simulink model "xobserver"  (R2018a)
settings: Solver=ode45  StartTime=0.0  StopTime=24.5344
model workspace (MAT data in the model file):
  control : struct (value not decoded)
  input : struct (value not decoded)
  l = 3335
  l1 = 2807
  l2 = 674
  lcontrol = 334
  lt = 665
  output : struct (value not decoded)
  output1 : struct (value not decoded)
  pitch = [-0.00601170594305 0.00114522514384 0.0125445164557 0.0260129427859 0.0413526501937 0.0511756269945 0.0373024628261 0.0532548324432 0.0752374412467 0.0870367972512 0.0703790408797 0.0642023494021 ... (665 elements, 665x1)]
  pitch1 = [0.00235222572609 0.0162413418271 0.0237914073903 0.038703711523 0.0528926975341 0.0693959637901 0.125700648169 0.149036541994 0.168586162345 0.181978559157 0.17648303704 0.173940572128 ... (665 elements, 665x1)]
  roll = [-0.00280308900026 -0.0093555701281 -0.00623960724973 -0.00965013944258 -0.0144960083544 -0.0165739618303 -0.0413451111402 -0.0417587932814 -0.039753610855 -0.0382742391951 -0.0474672160662 -0.0523524236581 ... (665 elements, 665x1)]
  roll1 = [-0.00508976540984 -0.0128769177256 -0.00573808802069 -0.00803683640664 -0.0148569990238 -0.0135250113299 0.00757283220458 0.0108108566268 0.0110824245139 0.0117467287189 0.0115391118445 0.00812049366445 ... (665 elements, 665x1)]
  rtk_P = [0 0 0.00725817699424 0.00725817699424 -4.192609801e-16 -4.192609801e-16 0.00725817698288 0.00725817698288 -6.06069014419e-17 -6.06069014419e-17 0.00725817697152 0.00725817697152 ... (2022 elements, 674x3)]
  simin : struct (value not decoded)
  t = [85.2681087899 153.847078989 135.937655107 145.710208503 139.738803374 143.646452387 141.245887466 142.795164057 141.986419874 142.477492231 142.340892456 142.389396391 ... (674 elements, 674x1)]
  temp = [0.000186264650653 -0.000333016556148 0.00127742410264 0.00224038281138 0.00429726594319 -0.00123745127094 -0.0498635877438 -0.0654781132175 -0.0797628012916 -0.0994190421594 -0.130389530625 -0.157448428987 ... (674 elements, 674x1)]
  time = [137013148 137105522 137113114 137205498 137213142 137305502 137313143 137385536 137393177 137505497 137513125 137605502 ... (665 elements, 665x1)]
  tout = [0 40 80 120 160 200 240 280 320 360 400 440 ... (51 elements, 51x1)]
  ups = [-0.00390798864963 -0.0343320965106 -0.0636578539957 -0.075087173802 -0.0805963166531 -0.0991310672402 -0.125807682301 -0.141612416937 -0.141039897482 -0.132345709554 -0.120718475957 -0.105525554245 ... (665 elements, 665x1)]
  urs = [-0.0193064957453 -0.00988556947443 0.00896900324588 0.0192245887848 0.0131872654637 -0.000864770461033 -0.0106332547779 -0.00981483295256 -0.00119475892361 0.00693320512295 0.00799889781381 0.00317561720843 ... (665 elements, 665x1)]
  uts = [0.664106860951 0.749481484877 0.672099541838 0.648171853238 0.700691335264 0.708512249166 0.659850468498 0.640879189244 0.664961763399 0.668205140062 0.640989688844 0.625700347079 ... (665 elements, 665x1)]
  uys = [0.0139395447601 0.0198481563309 0.0256425224772 0.0339606547853 0.0446716994275 0.0544470884218 0.06301463774 0.0718767917399 0.0826736407 0.0943232231429 0.10641126735 0.11853603151 ... (665 elements, 665x1)]
  x = [8.71560944851e-05 -0.000263895544732 0.000265805954332 0.000300014003894 0.000591371497193 0.000529778841884 0.00684193504836 0.00668914061072 0.00254694811157 -0.00143805981445 -0.0136823182856 -0.0178010839904 ... (665 elements, 665x1)]
  x1 = [8.54283814042e-05 -0.000351541918258 0.000561343727981 0.00122062991294 0.00226118745505 0.0017878063312 -0.0048216263535 -0.0106732543262 -0.0180693220189 -0.0278330591582 -0.0298109986026 -0.0413157469741 ... (665 elements, 665x1)]
  x_av = [8.62922379446e-05 -0.000307718731495 0.000413574841157 0.000760321958416 0.00142627947612 0.00115879258654 0.00101015434743 -0.00199205685772 -0.00776118695365 -0.0146355594863 -0.0217466584441 -0.0295584154823 ... (665 elements, 665x1)]
  xt = [-6.06069014419e-17 0.00725817697152 0.00725817697152 -5.47955244547e-11 -5.47955244547e-11 -5.57118682784e-11 -5.57118682784e-11 -0.00725817702815 -0.00725817702815 -0.0145163542274 -0.0145163542274 -0.0290327088019 ... (665 elements, 665x1)]
  y = [4.71199364932e-05 -0.000202451032641 0.00110205359743 0.00274075291804 0.00386317545071 0.0039759501557 0.0111320604636 0.0200674919449 0.0256167559869 0.0328388617799 0.00902856975366 0.0187732326011 ... (665 elements, 665x1)]
  y1 = [0.000186264650653 -0.000333016556148 0.00127742410264 0.00224038281138 0.00429726594319 -0.00123745127094 -0.0498635877438 -0.0654781132175 -0.0797628012916 -0.0994190421594 -0.130389530625 -0.157448428987 ... (665 elements, 665x1)]
  y_av = [0.000116692293573 -0.000267733794395 0.00118973885004 0.00249056786471 0.00408022069695 0.00136924944238 -0.0193657636401 -0.0227053106363 -0.0270730226523 -0.0332900901898 -0.0606804804357 -0.0693375981928 ... (665 elements, 665x1)]
  yaw = [0.551630744054 0.985953522054 0.860467849076 0.912170384354 0.864267212524 0.877979115519 0.85252446167 0.850917442274 0.835099319744 0.825993656962 0.8192363021 0.809230396231 ... (665 elements, 665x1)]
  yaw1 = [0.524311158471 0.914078236382 0.795656408279 0.841193934159 0.796803282272 0.809519389357 0.787366234758 0.785910630038 0.771945888619 0.763168855651 0.757543515422 0.745155737898 ... (665 elements, 665x1)]
  yt = [2.07646400074e-15 -8.22783768201e-10 -8.22783768201e-10 -0.0111218847698 -0.0111218847698 -0.0222437696223 -0.0222437696223 -0.0333656546197 -0.0333656546197 -0.0444875400883 -0.0444875400883 -0.0667313107556 ... (665 elements, 665x1)]
  z = [-0.0994666679592 -0.214162644666 -0.215226967159 -0.256145303395 -0.292239651406 -0.309925352113 -0.350361829325 -0.36096245045 -0.394865238248 -0.398678408621 -0.417742992449 -0.417553654594 ... (674 elements, 674x1)]
  z1 = [-0.103229820714 -0.203136396463 -0.194407590044 -0.247819005734 -0.277075354685 -0.291884441153 -0.321788426104 -0.334001860067 -0.367445284083 -0.368818531247 -0.415153871284 -0.416306471083 ... (674 elements, 674x1)]
libraries: dspmathops x3
(part 2 of 2)

== system xobserver/Norm 1 ==
  In1 : Inport
  In2 : Inport  Port=2
  Sqrt : Sqrt  SaturateOnIntegerOverflow=on
  Square : Math  Operator=square  SaturateOnIntegerOverflow=on
  Square1 : Math  Operator=square  SaturateOnIntegerOverflow=on
  Sum2 : Sum  Inputs=|++
  Out1 : Outport
  wires:
  Sum2/1 -> Sqrt/1
  Square1/1 -> Sum2/2
  Square/1 -> Sum2/1
  In2/1 -> Square1/1
  Sqrt/1 -> Out1/1
  In1/1 -> Square/1

== system xobserver/Norm 2 ==
  In1 : Inport
  In2 : Inport  Port=2
  Sqrt : Sqrt  SaturateOnIntegerOverflow=on
  Square : Math  Operator=square  SaturateOnIntegerOverflow=on
  Square1 : Math  Operator=square  SaturateOnIntegerOverflow=on
  Sum2 : Sum  Inputs=|++
  Out1 : Outport
  wires:
  Sum2/1 -> Sqrt/1
  Square1/1 -> Sum2/2
  Square/1 -> Sum2/1
  In2/1 -> Square1/1
  Sqrt/1 -> Out1/1
  In1/1 -> Square/1

== system xobserver/Norm 3 ==
  In1 : Inport
  In2 : Inport  Port=2
  Sqrt : Sqrt  SaturateOnIntegerOverflow=on
  Square : Math  Operator=square  SaturateOnIntegerOverflow=on
  Square1 : Math  Operator=square  SaturateOnIntegerOverflow=on
  Sum2 : Sum  Inputs=|++
  Out1 : Outport
  wires:
  Sum2/1 -> Sqrt/1
  Square1/1 -> Sum2/2
  Square/1 -> Sum2/1
  In2/1 -> Square1/1
  Sqrt/1 -> Out1/1
  In1/1 -> Square/1

== system xobserver/Norm 5 ==
  In1 : Inport
  In2 : Inport  Port=2
  Sqrt : Sqrt  SaturateOnIntegerOverflow=on
  Square : Math  Operator=square  SaturateOnIntegerOverflow=on
  Square1 : Math  Operator=square  SaturateOnIntegerOverflow=on
  Sum2 : Sum  Inputs=|++
  Out1 : Outport
  wires:
  Sum2/1 -> Sqrt/1
  Square1/1 -> Sum2/2
  Square/1 -> Sum2/1
  In2/1 -> Square1/1
  Sqrt/1 -> Out1/1
  In1/1 -> Square/1

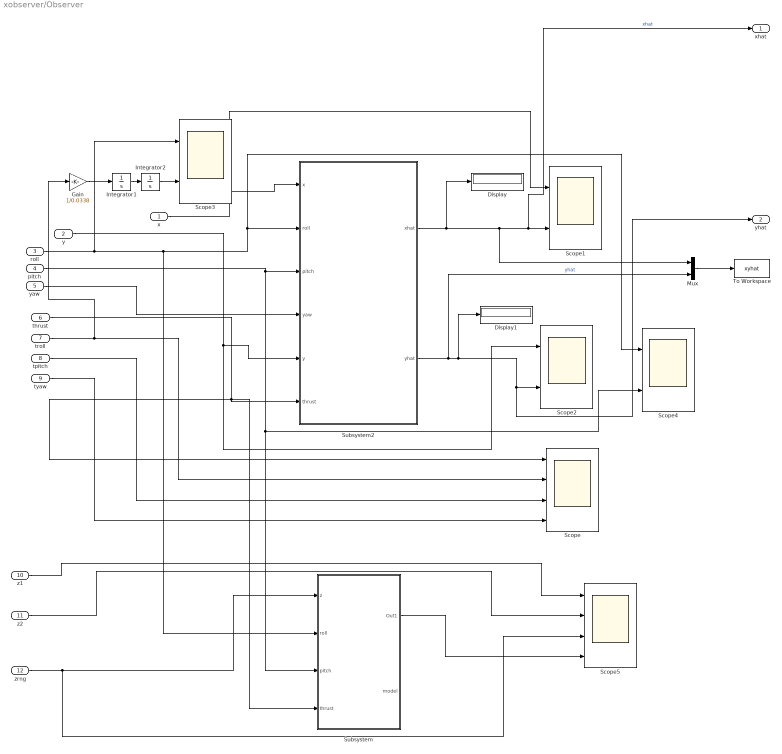
== system xobserver/Observer  ==
  x : Inport
  y : Inport  Port=2
  roll : Inport  Port=3
  pitch : Inport  Port=4
  yaw : Inport  Port=5
  thrust : Inport  Port=6
  troll : Inport  Port=7
  tpitch : Inport  Port=8
  tyaw : Inport  Port=9
  z1 : Inport  Port=10
  z2 : Inport  Port=11
  "zrng " : Inport  Port=12
  Display : Display
  Display1 : Display
  Gain : Gain  Gain=1/0.0338
  Integrator1 : Integrator
  Integrator2 : Integrator
  Mux : Mux  Inputs=2
  Scope : Scope  NumInputPorts=4
  Scope{1..4} (4 alike) : Scope  NumInputPorts=2
  Scope5 : Scope  NumInputPorts=4
  Subsystem : Subsystem
  Subsystem2 : Subsystem
  To Workspace : ToWorkspace  VariableName=xyhat  SampleTime=0.01
  xhat : Outport
  yhat : Outport  Port=2
  wires:
  y/1 -> Subsystem2/5(y), Scope2/1
  pitch/1 -> Scope4/2, Subsystem/3(pitch), Subsystem2/3(pitch)
  tyaw/1 -> Scope/4
  Subsystem2/2(yhat) -> Mux/2, Display1/1, yhat/1, Scope2/2  "yhat"
  thrust/1 -> Scope/1, Subsystem2/6(thrust), Subsystem/4(thrust)
  roll/1 -> Scope4/1, Subsystem2/2(roll), Subsystem/2(roll), Scope3/1
  troll/1 -> Gain/1, Scope/2
  Mux/1 -> To Workspace/1
  x/1 -> Subsystem2/1(x), Scope1/1
  yaw/1 -> Subsystem2/4(yaw)
  tpitch/1 -> Scope/3
  Gain/1 -> Integrator1/1
  Integrator1/1 -> Integrator2/1
  Integrator2/1 -> Scope3/2
  Subsystem2/1(xhat) -> Display/1, xhat/1, Scope1/2, Mux/1  "xhat"
  z1/1 -> Scope5/1
  z2/1 -> Scope5/2
  "zrng "/1 -> Subsystem/1(z), Scope5/3
  Subsystem/1(Out1) -> Scope5/4

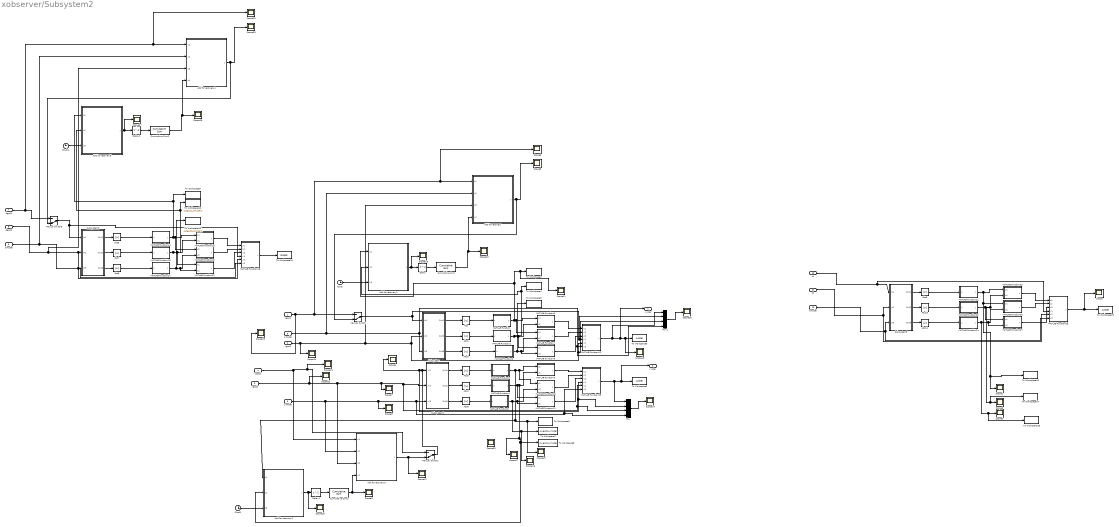
== system xobserver/Subsystem2 ==
  "xgps1 " : Inport
  "xgps2 " : Inport  Port=2
  "ygps2 " : Inport  Port=3
  ygps1 : Inport  Port=4
  "xmodel " : Inport  Port=5
  "ymodel " : Inport  Port=6
  "dgps1 " : Inport  Port=7
  dgps2 : Inport  Port=8
  "dmodel " : Inport  Port=9
  "z1 " : Inport  Port=10
  z2 : Inport  Port=11
  "zmodel " : Inport  Port=12
  Abs{,1..11} (12 alike) : Abs
  Add for recovery : MATLAB Function  TreatAsAtomicUnit=on
  Add for recovery1 : MATLAB Function  TreatAsAtomicUnit=on
  Add for recovery2 : MATLAB Function  TreatAsAtomicUnit=on
  Add for recovery3 : MATLAB Function  TreatAsAtomicUnit=on
  Add for recovery4 : MATLAB Function  TreatAsAtomicUnit=on
  Add for recovery5 : MATLAB Function  TreatAsAtomicUnit=on
  Clock : Clock
  Clock1 : Clock
  Clock2 : Clock
  Cumulative Sum : dspmathops/Cumulative Sum  dim=Channels (running sum)  InputProcessing=Columns as channels (frame based)  reset_popup=None  roundingMode=Floor  overflowMode=off  outputDataTypeStr=Inherit: Same as accumulator  outputMin=[]  outputMax=[]  outputLastDataTypeStr=Inherit: Same as accumulator
      settings: SourceProductName=DSP System Toolbox
  Cumulative Sum1 : dspmathops/Cumulative Sum  dim=Channels (running sum)  InputProcessing=Columns as channels (frame based)  reset_popup=None  roundingMode=Floor  overflowMode=off  outputDataTypeStr=Inherit: Same as accumulator  outputMin=[]  outputMax=[]  outputLastDataTypeStr=Inherit: Same as accumulator
      settings: SourceProductName=DSP System Toolbox
  Cumulative Sum2 : dspmathops/Cumulative Sum  dim=Channels (running sum)  InputProcessing=Columns as channels (frame based)  reset_popup=None  roundingMode=Floor  overflowMode=off  outputDataTypeStr=Inherit: Same as accumulator  outputMin=[]  outputMax=[]  outputLastDataTypeStr=Inherit: Same as accumulator
      settings: SourceProductName=DSP System Toolbox
  Delay : Delay
  Delay1 : Delay
  Delay2 : Delay
  MATLAB Function : MATLAB Function  TreatAsAtomicUnit=on
  MATLAB Function1 : MATLAB Function  TreatAsAtomicUnit=on
  MATLAB Function10 : MATLAB Function  TreatAsAtomicUnit=on
  MATLAB Function11 : MATLAB Function  TreatAsAtomicUnit=on
  MATLAB Function12 : MATLAB Function  TreatAsAtomicUnit=on
  MATLAB Function13 : MATLAB Function  TreatAsAtomicUnit=on
  MATLAB Function14 : MATLAB Function  TreatAsAtomicUnit=on
  MATLAB Function15 : MATLAB Function  TreatAsAtomicUnit=on
  MATLAB Function16 : MATLAB Function  TreatAsAtomicUnit=on
  MATLAB Function17 : MATLAB Function  TreatAsAtomicUnit=on
  MATLAB Function18 : MATLAB Function  TreatAsAtomicUnit=on
  MATLAB Function19 : MATLAB Function  TreatAsAtomicUnit=on
  MATLAB Function2 : MATLAB Function  TreatAsAtomicUnit=on
  MATLAB Function20 : MATLAB Function  TreatAsAtomicUnit=on
  MATLAB Function21 : MATLAB Function  TreatAsAtomicUnit=on
  MATLAB Function22 : MATLAB Function  TreatAsAtomicUnit=on
  MATLAB Function23 : MATLAB Function  TreatAsAtomicUnit=on
  MATLAB Function24 : MATLAB Function  TreatAsAtomicUnit=on
  MATLAB Function25 : MATLAB Function  TreatAsAtomicUnit=on
  MATLAB Function26 : MATLAB Function  TreatAsAtomicUnit=on
  MATLAB Function27 : MATLAB Function  TreatAsAtomicUnit=on
  MATLAB Function3 : MATLAB Function  TreatAsAtomicUnit=on
  MATLAB Function4 : MATLAB Function  TreatAsAtomicUnit=on
  MATLAB Function5 : MATLAB Function  TreatAsAtomicUnit=on
  MATLAB Function6 : MATLAB Function  TreatAsAtomicUnit=on
  MATLAB Function7 : MATLAB Function  TreatAsAtomicUnit=on
  MATLAB Function8 : MATLAB Function  TreatAsAtomicUnit=on
  MATLAB Function9 : MATLAB Function  TreatAsAtomicUnit=on
  Manual Switch : ManualSwitch  CurrentSetting=0
  Manual Switch1 : ManualSwitch  CurrentSetting=0
  Manual Switch3 : ManualSwitch  CurrentSetting=0
  Mux : Mux
  Mux1 : Mux
  Scope{,1..29} (30 alike) : Scope
  Subsystem : Subsystem
  Subsystem1 : Subsystem
  Subsystem2 : Subsystem
  Subsystem3 : Subsystem
  To Workspace1 : ToWorkspace  VariableName=yvoter  SampleTime=0.01
  To Workspace10 : ToWorkspace  VariableName=dvoter  SampleTime=0.01
  To Workspace11 : ToWorkspace  VariableName=s_dgps1_dmodel1  SampleTime=-1
  To Workspace12 : ToWorkspace  VariableName=s_dgps2_dmodel1  SampleTime=-1
  To Workspace13 : ToWorkspace  VariableName=zvoter  SampleTime=0.01
  To Workspace14 : ToWorkspace  VariableName=s_zrng1_zmodel  SampleTime=-1
  To Workspace15 : ToWorkspace  VariableName=s_zrng2_zmodel  SampleTime=-1
  To Workspace16 : ToWorkspace  VariableName=s_zrng1_zrng2  SampleTime=-1
  To Workspace2 : ToWorkspace  VariableName=s_xgps1_xgps2  SampleTime=-1
  To Workspace3 : ToWorkspace  VariableName=xvoter  SampleTime=0.01
  To Workspace4 : ToWorkspace  VariableName=s_xgps1_xmodel  SampleTime=-1
  To Workspace5 : ToWorkspace  VariableName=s_xgps2_xmodel  SampleTime=-1
  To Workspace6 : ToWorkspace  VariableName=s_ygps1_ygps2  SampleTime=-1
  To Workspace7 : ToWorkspace  VariableName=s_ygps2_ymodel  SampleTime=-1
  To Workspace8 : ToWorkspace  VariableName=s_ygps1_ymodel  SampleTime=-1
  To Workspace9 : ToWorkspace  VariableName=s_dgps1_dgps2  SampleTime=-1
  "xvoter " : Outport
  yvoter : Outport  Port=2
  wires:
  Subsystem/1(Out1) -> Abs/1
  Subsystem/3(Out3) -> Abs2/1
  "ymodel "/1 -> Add for recovery3/2(u2), Scope8/1, Subsystem1/3(In3), Mux/4, MATLAB Function13/6(x3)
  MATLAB Function9/1(y) -> MATLAB Function13/1(u1)
  MATLAB Function11/1(y) -> MATLAB Function13/3(u3)
  Manual Switch1/1 -> Scope4/1, Mux/2, MATLAB Function13/4(x1), Subsystem1/1(In1)
  Subsystem/2(Out2) -> Abs1/1
  Subsystem1/3(Out3) -> Abs5/1
  MATLAB Function4/1(y) -> Scope17/1, Add for recovery2/2(u2), To Workspace8/1, MATLAB Function9/2(u2), MATLAB Function11/1(u1)
  "xgps2 "/1 -> Scope24/1, Subsystem/2(In2), Mux1/3, MATLAB Function12/5(x2), Add for recovery/3(u3)
  MATLAB Function/1(y) -> Add for recovery1/1(u1), Scope11/1, To Workspace2/1, MATLAB Function7/1(u1), MATLAB Function6/1(u1)
  MATLAB Function2/1(y) -> To Workspace5/1, MATLAB Function8/2(u2), MATLAB Function7/2(u2)
  MATLAB Function13/1(y) -> Mux/1, yvoter/1, To Workspace1/1
  MATLAB Function5/1(y) -> MATLAB Function10/2(u2), MATLAB Function11/2(u2), Scope16/1, To Workspace7/1
  MATLAB Function3/1(y) -> Add for recovery2/1(u1), Scope15/1, To Workspace6/1, MATLAB Function10/1(u1), MATLAB Function9/1(u1)
  Manual Switch/1 -> Mux1/2, MATLAB Function12/4(x1), Subsystem/1(In1)
  MATLAB Function12/1(y) -> Mux1/1, "xvoter "/1, Scope13/1, To Workspace3/1
  MATLAB Function8/1(y) -> MATLAB Function12/3(u3)
  MATLAB Function1/1(y) -> Add for recovery1/2(u2), To Workspace4/1, MATLAB Function8/1(u1), MATLAB Function6/2(u2)
  "xmodel "/1 -> Add for recovery/2(u2), Subsystem/3(In3), Mux1/4, MATLAB Function12/6(x3)
  MATLAB Function7/1(y) -> MATLAB Function12/2(u2)
  MATLAB Function6/1(y) -> MATLAB Function12/1(u1)
  "ygps2 "/1 -> Scope22/1, Add for recovery3/3(u3), Scope7/1, Subsystem1/2(In2), Mux/3, MATLAB Function13/5(x2)
  Subsystem1/1(Out1) -> Abs3/1
  Subsystem1/2(Out2) -> Abs4/1
  MATLAB Function10/1(y) -> MATLAB Function13/2(u2)
  MATLAB Function18/1(y) -> MATLAB Function16/1(u1)
  MATLAB Function19/1(y) -> MATLAB Function16/2(u2)
  MATLAB Function16/1(y) -> To Workspace10/1
  MATLAB Function20/1(y) -> MATLAB Function16/3(u3)
  MATLAB Function15/1(y) -> Add for recovery5/2(u2), To Workspace11/1, MATLAB Function20/1(u1), MATLAB Function18/2(u2)
  MATLAB Function14/1(y) -> Add for recovery5/1(u1), To Workspace9/1, MATLAB Function19/1(u1), MATLAB Function18/1(u1)
  MATLAB Function17/1(y) -> To Workspace12/1, MATLAB Function20/2(u2), MATLAB Function19/2(u2)
  Subsystem2/1(Out1) -> Abs6/1
  Subsystem2/2(Out2) -> Abs7/1
  Subsystem2/3(Out3) -> Abs8/1
  Abs/1 -> MATLAB Function/1(u)
  Abs1/1 -> MATLAB Function1/1(u)
  Abs2/1 -> MATLAB Function2/1(u)
  Abs3/1 -> MATLAB Function3/1(u)
  Abs4/1 -> MATLAB Function4/1(u)
  Abs5/1 -> MATLAB Function5/1(u)
  Abs6/1 -> MATLAB Function14/1(u)
  Abs7/1 -> MATLAB Function15/1(u)
  Abs8/1 -> MATLAB Function17/1(u)
  MATLAB Function21/1(y) -> To Workspace16/1, Scope1/1, MATLAB Function26/1(u1), MATLAB Function25/1(u1)
  MATLAB Function24/1(y) -> To Workspace15/1, Scope3/1, MATLAB Function27/2(u2), MATLAB Function26/2(u2)
  Abs10/1 -> MATLAB Function22/1(u)
  Abs11/1 -> MATLAB Function24/1(u)
  Abs9/1 -> MATLAB Function21/1(u)
  MATLAB Function25/1(y) -> MATLAB Function23/1(u1)
  Subsystem3/2(Out2) -> Abs10/1
  MATLAB Function26/1(y) -> MATLAB Function23/2(u2)
  Subsystem3/1(Out1) -> Abs9/1
  MATLAB Function23/1(y) -> Scope/1, To Workspace13/1
  MATLAB Function27/1(y) -> MATLAB Function23/3(u3)
  MATLAB Function22/1(y) -> To Workspace14/1, Scope2/1, MATLAB Function25/2(u2), MATLAB Function27/1(u1)
  Subsystem3/3(Out3) -> Abs11/1
  "xgps1 "/1 -> Scope23/1, Scope6/1, Add for recovery/1(u1), Manual Switch/1
  Clock/1 -> Add for recovery1/3(u3)
  Clock1/1 -> Add for recovery2/3(u3)
  ygps1/1 -> Scope21/1, Manual Switch1/1, Add for recovery3/1(u1)
  Add for recovery1/1(y) -> Scope19/1, Delay/1
  Cumulative Sum/1 -> Add for recovery/4(u4), Scope10/1
  Delay/1 -> Cumulative Sum/1
  Delay1/1 -> Cumulative Sum1/1
  Add for recovery2/1(y) -> Scope18/1, Delay1/1
  Cumulative Sum1/1 -> Add for recovery3/4(u4), Scope9/1
  Add for recovery3/1(y) -> Scope12/1, Manual Switch1/2
  Add for recovery/1(y) -> Manual Switch/2, Scope5/1
  Mux/1 -> Scope14/1
  Mux1/1 -> Scope20/1
  z2/1 -> MATLAB Function23/5(x2), Subsystem3/2(In2)
  "zmodel "/1 -> MATLAB Function23/6(x3), Subsystem3/3(In3)
  "z1 "/1 -> MATLAB Function23/4(x1), Subsystem3/1(In1)
  dgps2/1 -> Add for recovery4/3(u3), MATLAB Function16/5(x2), Subsystem2/2(In2)
  "dmodel "/1 -> Add for recovery4/2(u2), MATLAB Function16/6(x3), Subsystem2/3(In3)
  "dgps1 "/1 -> Scope29/1, Add for recovery4/1(u1), Manual Switch3/1
  Add for recovery4/1(y) -> Manual Switch3/2, Scope28/1
  Cumulative Sum2/1 -> Add for recovery4/4(u4), Scope26/1
  Add for recovery5/1(y) -> Scope27/1, Delay2/1
  Delay2/1 -> Cumulative Sum2/1
  Clock2/1 -> Add for recovery5/3(u3)
  Manual Switch3/1 -> MATLAB Function16/4(x1), Subsystem2/1(In1)

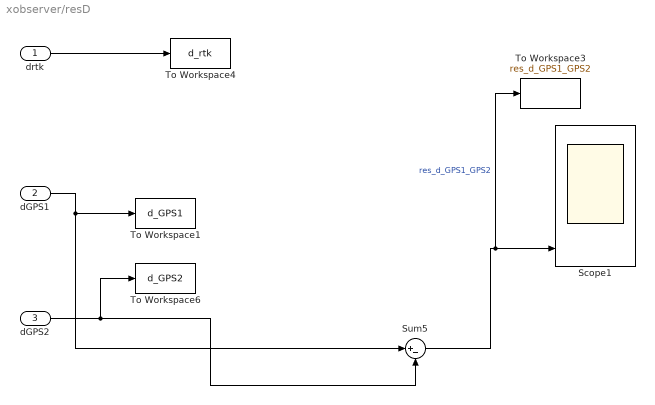
== system xobserver/resD ==
  drtk : Inport
  dGPS1 : Inport  Port=2
  dGPS2 : Inport  Port=3
  Scope1 : Scope  NumInputPorts=4
  Sum5 : Sum  Inputs=|+-
  To Workspace1 : ToWorkspace  VariableName=d_GPS1  SampleTime=0.01
  To Workspace3 : ToWorkspace  VariableName=res_d_GPS1_GPS2  SampleTime=0.01
  To Workspace4 : ToWorkspace  VariableName=d_rtk  SampleTime=0.01
  To Workspace6 : ToWorkspace  VariableName=d_GPS2  SampleTime=0.01
  wires:
  Sum5/1 -> To Workspace3/1, Scope1/4  "res_d_GPS1_GPS2"
  dGPS2/1 -> To Workspace6/1, Sum5/2
  drtk/1 -> To Workspace4/1
  dGPS1/1 -> To Workspace1/1, Sum5/1

== system xobserver/resD1 ==
  xrtk : Inport
  xGPS1 : Inport  Port=2
  xGPS2 : Inport  Port=3
  Scope1 : Scope  NumInputPorts=4
  Sum5 : Sum  Inputs=|+-
  To Workspace3 : ToWorkspace  VariableName=res_x_GPS1_GPS2  SampleTime=0.01
  wires:
  xGPS1/1 -> Sum5/1
  xGPS2/1 -> Sum5/2
  Sum5/1 -> To Workspace3/1, Scope1/4  "res_x_GPS1_GPS2"

== system xobserver/resD2 ==
  yrtk : Inport
  yGPS1 : Inport  Port=2
  yGPS2 : Inport  Port=3
  Scope1 : Scope  NumInputPorts=4
  Sum5 : Sum  Inputs=|+-
  To Workspace3 : ToWorkspace  VariableName=res_y_GPS1_GPS2  SampleTime=0.01
  wires:
  yGPS1/1 -> Sum5/1
  Sum5/1 -> To Workspace3/1, Scope1/4  "res_y_GPS1_GPS2"
  yGPS2/1 -> Sum5/2

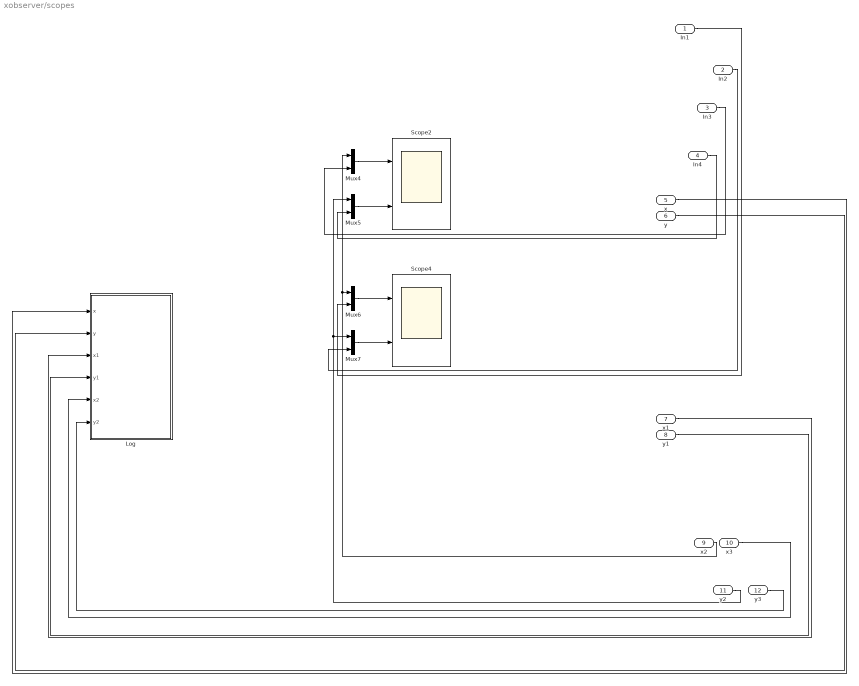
== system xobserver/scopes  ==
  In1 : Inport
  In2 : Inport  Port=2
  In3 : Inport  Port=3
  In4 : Inport  Port=4
  x : Inport  Port=5
  y : Inport  Port=6
  x1 : Inport  Port=7
  y1 : Inport  Port=8
  x2 : Inport  Port=9
  x3 : Inport  Port=10
  y2 : Inport  Port=11
  y3 : Inport  Port=12
  "Log " : Subsystem
  Mux{4..7} (4 alike) : Mux  Inputs=2
  Scope2 : Scope  NumInputPorts=2
  Scope4 : Scope  NumInputPorts=2
  wires:
  In3/1 -> Mux4/2
  In1/1 -> Mux6/2
  y1/1 -> "Log "/4(y1)
  Mux7/1 -> Scope4/2
  y2/1 -> Mux7/1, Mux5/1
  Mux6/1 -> Scope4/1
  Mux5/1 -> Scope2/2
  Mux4/1 -> Scope2/1
  x2/1 -> Mux6/1, Mux4/1
  In2/1 -> Mux7/2
  In4/1 -> Mux5/2
  y/1 -> "Log "/2(y)
  x/1 -> "Log "/1(x)
  x1/1 -> "Log "/3(x1)
  y3/1 -> "Log "/6(y2)
  x3/1 -> "Log "/5(x2)

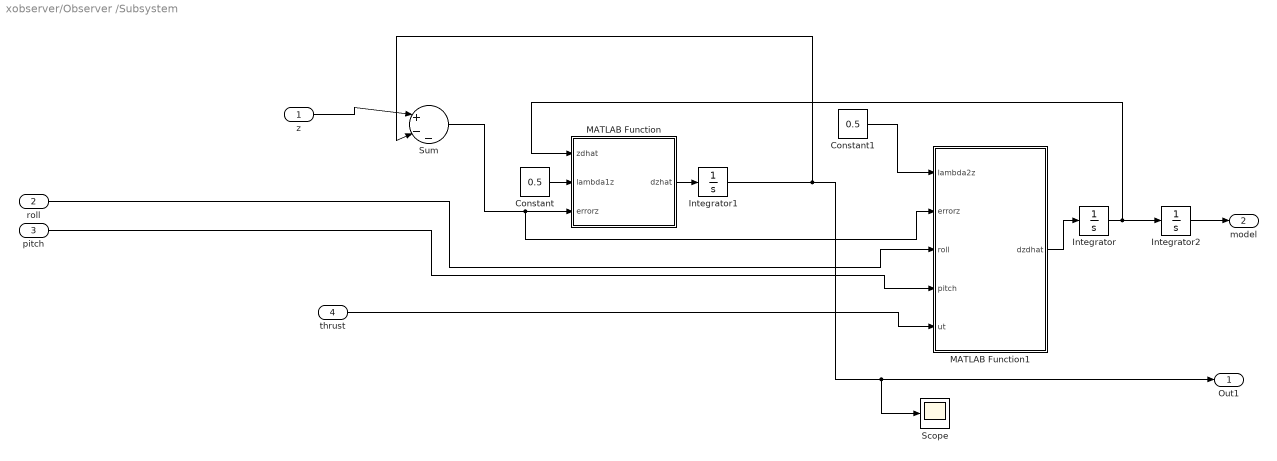
== system xobserver/Observer /Subsystem ==
  z : Inport
  roll : Inport  Port=2
  pitch : Inport  Port=3
  thrust : Inport  Port=4
  Constant : Constant  Value=0.5
  Constant1 : Constant  Value=0.5
  Integrator : Integrator  InitialCondition=0
  Integrator1 : Integrator  InitialCondition=0.1332
  Integrator2 : Integrator
  MATLAB Function : MATLAB Function  TreatAsAtomicUnit=on
  MATLAB Function1 : MATLAB Function  TreatAsAtomicUnit=on
  Scope : Scope
  Sum : Sum  Inputs=|+--
  Out1 : Outport
  "model " : Outport  Port=2
  wires:
  MATLAB Function/1(dzhat) -> Integrator1/1
  Integrator/1 -> Integrator2/1, MATLAB Function/1(zdhat)
  Constant1/1 -> MATLAB Function1/1(lambda2z)
  roll/1 -> MATLAB Function1/3(roll)
  Constant/1 -> MATLAB Function/2(lambda1z)
  MATLAB Function1/1(dzdhat) -> Integrator/1
  pitch/1 -> MATLAB Function1/4(pitch)
  thrust/1 -> MATLAB Function1/5(ut)
  z/1 -> Sum/1
  Integrator2/1 -> "model "/1
  Sum/1 -> MATLAB Function1/2(errorz), MATLAB Function/3(errorz)
  Integrator1/1 -> Sum/2, Scope/1, Out1/1

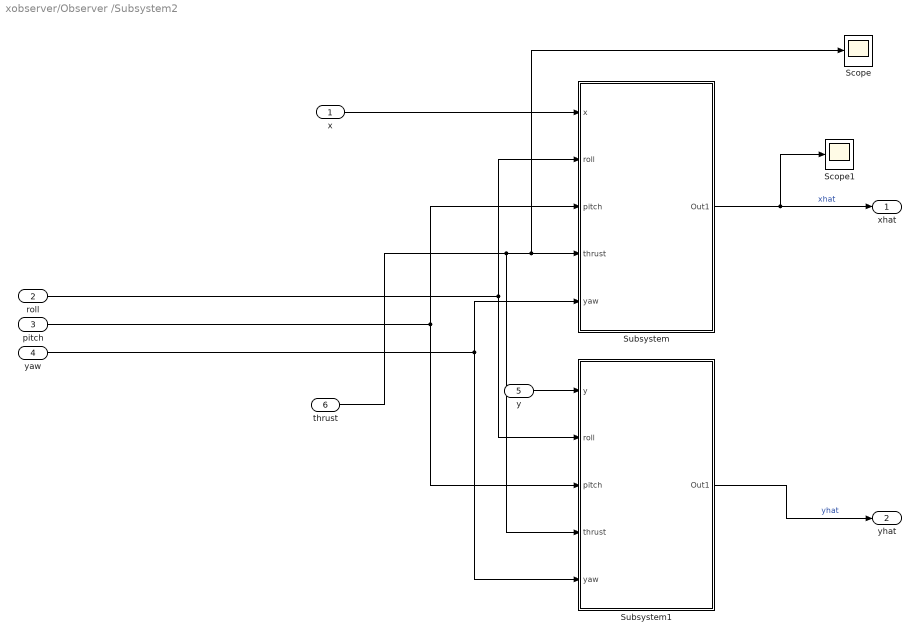
== system xobserver/Observer /Subsystem2 ==
  x : Inport
  roll : Inport  Port=2
  pitch : Inport  Port=3
  yaw : Inport  Port=4
  y : Inport  Port=5
  thrust : Inport  Port=6
  Scope : Scope
  Scope1 : Scope
  Subsystem : Subsystem
  Subsystem1 : Subsystem
  xhat : Outport
  yhat : Outport  Port=2
  wires:
  x/1 -> Subsystem/1(x)
  pitch/1 -> Subsystem/3(pitch), Subsystem1/3(pitch)
  yaw/1 -> Subsystem/5(yaw), Subsystem1/5(yaw)
  Subsystem/1(Out1) -> Scope1/1, xhat/1  "xhat"
  y/1 -> Subsystem1/1(y)
  roll/1 -> Subsystem/2(roll), Subsystem1/2(roll)
  thrust/1 -> Subsystem1/4(thrust), Scope/1, Subsystem/4(thrust)
  Subsystem1/1(Out1) -> yhat/1  "yhat"

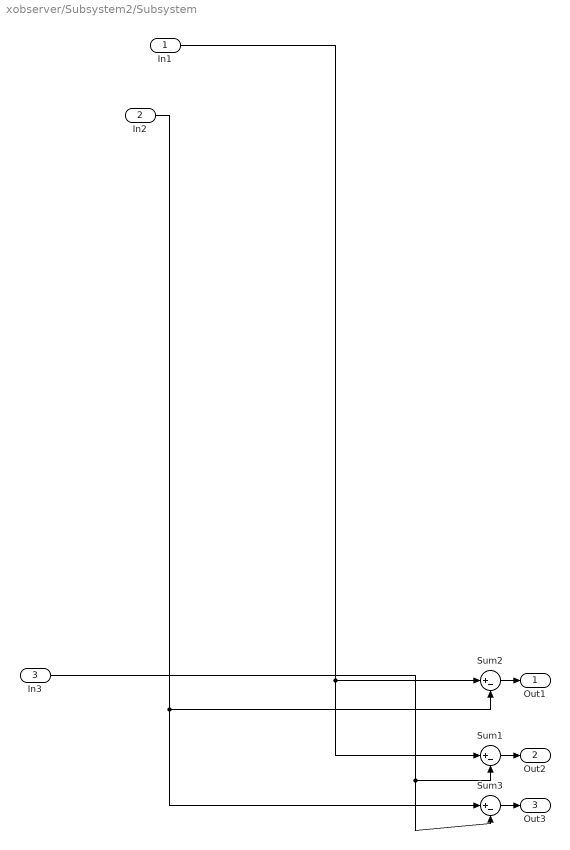
== system xobserver/Subsystem2/Subsystem ==
  In1 : Inport
  In2 : Inport  Port=2
  In3 : Inport  Port=3
  Sum1 : Sum  Inputs=|+-
  Sum2 : Sum  Inputs=|+-
  Sum3 : Sum  Inputs=|+-
  Out1 : Outport
  Out2 : Outport  Port=2
  Out3 : Outport  Port=3
  wires:
  Sum3/1 -> Out3/1
  In3/1 -> Sum3/2, Sum1/2
  Sum2/1 -> Out1/1
  In2/1 -> Sum2/2, Sum3/1
  In1/1 -> Sum2/1, Sum1/1
  Sum1/1 -> Out2/1

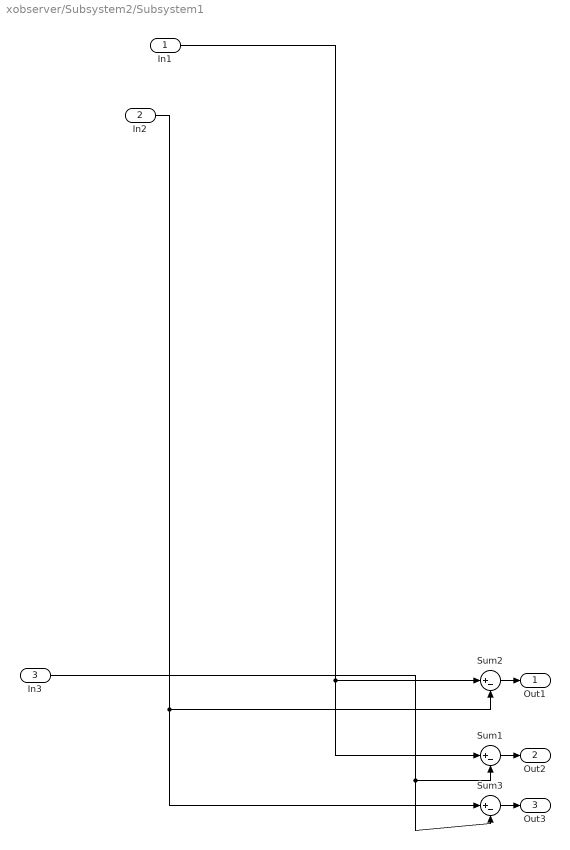
== system xobserver/Subsystem2/Subsystem1 ==
  In1 : Inport
  In2 : Inport  Port=2
  In3 : Inport  Port=3
  Sum1 : Sum  Inputs=|+-
  Sum2 : Sum  Inputs=|+-
  Sum3 : Sum  Inputs=|+-
  Out1 : Outport
  Out2 : Outport  Port=2
  Out3 : Outport  Port=3
  wires:
  Sum3/1 -> Out3/1
  In3/1 -> Sum3/2, Sum1/2
  Sum2/1 -> Out1/1
  In2/1 -> Sum2/2, Sum3/1
  In1/1 -> Sum2/1, Sum1/1
  Sum1/1 -> Out2/1

== system xobserver/Subsystem2/Subsystem2 ==
  In1 : Inport
  In2 : Inport  Port=2
  In3 : Inport  Port=3
  Sum1 : Sum  Inputs=|+-
  Sum2 : Sum  Inputs=|+-
  Sum3 : Sum  Inputs=|+-
  Out1 : Outport
  Out2 : Outport  Port=2
  Out3 : Outport  Port=3
  wires:
  Sum3/1 -> Out3/1
  In3/1 -> Sum3/2, Sum1/2
  Sum2/1 -> Out1/1
  In2/1 -> Sum2/2, Sum3/1
  In1/1 -> Sum2/1, Sum1/1
  Sum1/1 -> Out2/1

== system xobserver/Subsystem2/Subsystem3 ==
  In1 : Inport
  In2 : Inport  Port=2
  In3 : Inport  Port=3
  Sum1 : Sum  Inputs=|+-
  Sum2 : Sum  Inputs=|+-
  Sum3 : Sum  Inputs=|+-
  Out1 : Outport
  Out2 : Outport  Port=2
  Out3 : Outport  Port=3
  wires:
  Sum3/1 -> Out3/1
  In3/1 -> Sum3/2, Sum1/2
  Sum2/1 -> Out1/1
  In2/1 -> Sum2/2, Sum3/1
  In1/1 -> Sum2/1, Sum1/1
  Sum1/1 -> Out2/1

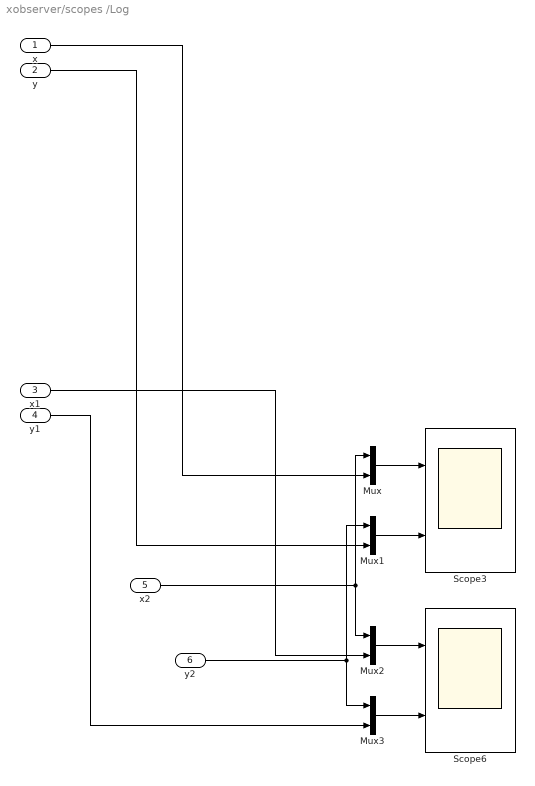
== system xobserver/scopes /Log  ==
  x : Inport
  y : Inport  Port=2
  x1 : Inport  Port=3
  y1 : Inport  Port=4
  x2 : Inport  Port=5
  y2 : Inport  Port=6
  Mux{,1..3} (4 alike) : Mux  Inputs=2
  Scope3 : Scope  NumInputPorts=2
  Scope6 : Scope  NumInputPorts=2
  wires:
  x1/1 -> Mux2/2
  y/1 -> Mux1/2
  Mux2/1 -> Scope6/1
  x2/1 -> Mux/1, Mux2/1
  Mux/1 -> Scope3/1
  Mux3/1 -> Scope6/2
  y1/1 -> Mux3/2
  y2/1 -> Mux1/1, Mux3/1
  Mux1/1 -> Scope3/2
  x/1 -> Mux/2

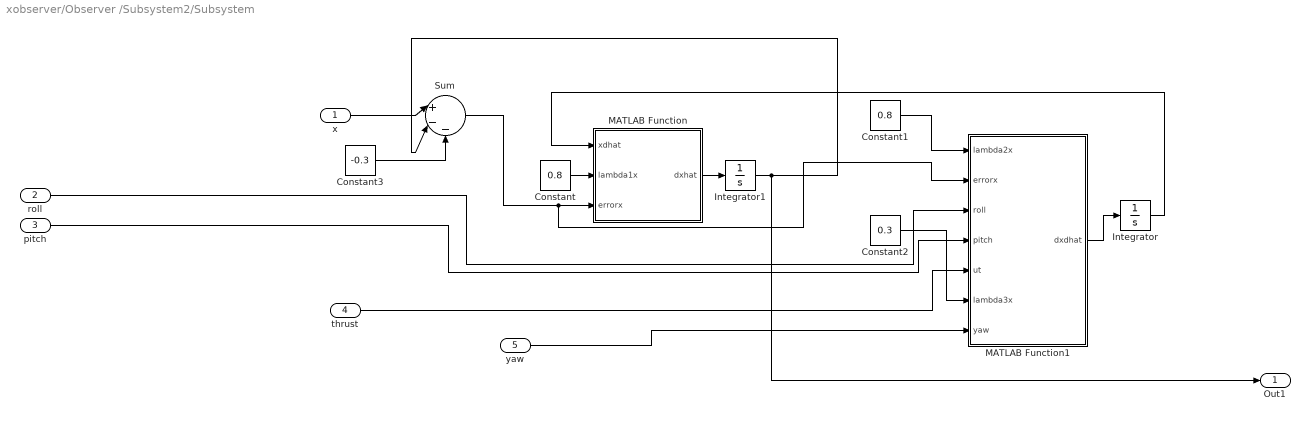
== system xobserver/Observer /Subsystem2/Subsystem ==
  x : Inport
  roll : Inport  Port=2
  pitch : Inport  Port=3
  thrust : Inport  Port=4
  yaw : Inport  Port=5
  Constant : Constant  Value=0.8
  Constant1 : Constant  Value=0.8
  Constant2 : Constant  Value=0.3
  Constant3 : Constant  Value=-0.3
  Integrator : Integrator
  Integrator1 : Integrator
  MATLAB Function : MATLAB Function  TreatAsAtomicUnit=on
  MATLAB Function1 : MATLAB Function  TreatAsAtomicUnit=on
  Sum : Sum  Inputs=|+--
  Out1 : Outport
  wires:
  Sum/1 -> MATLAB Function1/2(errorx), MATLAB Function/3(errorx)
  Integrator1/1 -> Out1/1, Sum/2
  MATLAB Function/1(dxhat) -> Integrator1/1
  Integrator/1 -> MATLAB Function/1(xdhat)
  Constant2/1 -> MATLAB Function1/6(lambda3x)
  Constant1/1 -> MATLAB Function1/1(lambda2x)
  roll/1 -> MATLAB Function1/3(roll)
  Constant/1 -> MATLAB Function/2(lambda1x)
  MATLAB Function1/1(dxdhat) -> Integrator/1
  pitch/1 -> MATLAB Function1/4(pitch)
  yaw/1 -> MATLAB Function1/7(yaw)
  thrust/1 -> MATLAB Function1/5(ut)
  x/1 -> Sum/1
  Constant3/1 -> Sum/3

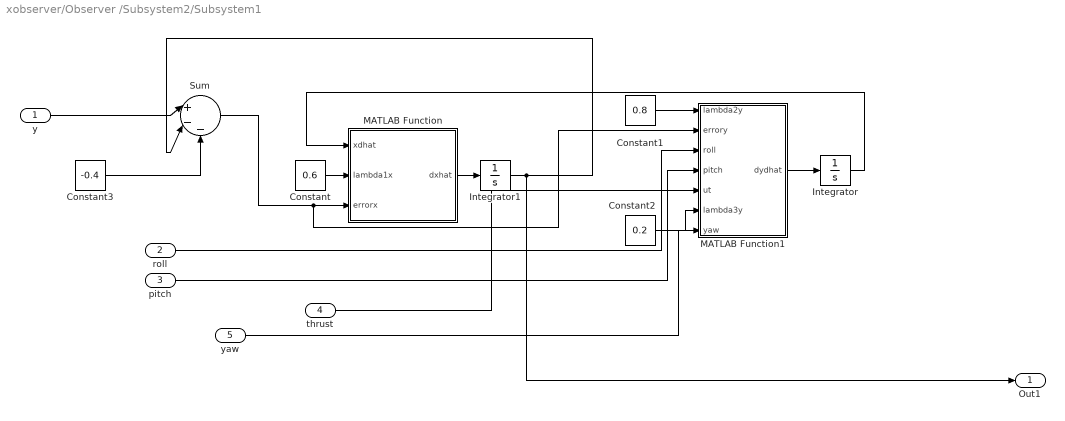
== system xobserver/Observer /Subsystem2/Subsystem1 ==
  y : Inport
  roll : Inport  Port=2
  pitch : Inport  Port=3
  thrust : Inport  Port=4
  yaw : Inport  Port=5
  Constant : Constant  Value=0.6
  Constant1 : Constant  Value=0.8
  Constant2 : Constant  Value=0.2
  Constant3 : Constant  Value=-0.4
  Integrator : Integrator
  Integrator1 : Integrator
  MATLAB Function : MATLAB Function  TreatAsAtomicUnit=on
  MATLAB Function1 : MATLAB Function  TreatAsAtomicUnit=on
  Sum : Sum  Inputs=|+--
  Out1 : Outport
  wires:
  Sum/1 -> MATLAB Function1/2(errory), MATLAB Function/3(errorx)
  Integrator1/1 -> Out1/1, Sum/2
  MATLAB Function/1(dxhat) -> Integrator1/1
  Integrator/1 -> MATLAB Function/1(xdhat)
  Constant2/1 -> MATLAB Function1/6(lambda3y)
  Constant1/1 -> MATLAB Function1/1(lambda2y)
  Constant/1 -> MATLAB Function/2(lambda1x)
  MATLAB Function1/1(dydhat) -> Integrator/1
  thrust/1 -> MATLAB Function1/5(ut)
  yaw/1 -> MATLAB Function1/7(yaw)
  pitch/1 -> MATLAB Function1/4(pitch)
  roll/1 -> MATLAB Function1/3(roll)
  y/1 -> Sum/1
  Constant3/1 -> Sum/3

== matlab function xobserver/Observer /Subsystem2/Subsystem/MATLAB Function1 ==
  data: lambda2x input; dxdhat output; errorx input; roll input; pitch input; ut input; lambda3x input; yaw input
function dxdhat = fcn(lambda2x, errorx, roll, pitch, ut, lambda3x, yaw)

dxdhat = (lambda3x*sign(errorx) + lambda2x*power(abs(errorx),2/3)*sign(errorx) - (cos(roll)*sin(pitch)*cos(yaw) + sin(roll)*sin(yaw))*ut)/1.6 ;
%%dxdhat = -(cos(roll)*sin(pitch)*cos(yaw) + sin(roll)*sin(yaw))*ut/1.8;

== matlab function xobserver/Observer /Subsystem2/Subsystem/MATLAB Function ==
  data: xdhat input; dxhat output; lambda1x input; errorx input
function dxhat = fcn(xdhat, lambda1x, errorx)

dxhat = xdhat + lambda1x*power(abs(errorx),2/3)*sign(errorx);
%%dxhat = xdhat;

== matlab function xobserver/Observer /Subsystem2/Subsystem1/MATLAB Function ==
  data: xdhat input; dxhat output; lambda1x input; errorx input
function dxhat = fcn(xdhat, lambda1x, errorx)

dxhat = xdhat + lambda1x*power(abs(errorx),2/3)*sign(errorx);

== matlab function xobserver/Observer /Subsystem2/Subsystem1/MATLAB Function1 ==
  data: lambda2y input; dydhat output; errory input; roll input; pitch input; ut input; lambda3y input; yaw input
function dydhat = fcn(lambda2y, errory, roll, pitch, ut, lambda3y, yaw)

dydhat =( lambda3y*sign(errory) + lambda2y*power(abs(errory),2/3)*sign(errory) - (cos(roll)*sin(pitch)*sin(yaw)-sin(roll)*cos(yaw))*ut)/1.6 ;

== matlab function xobserver/Subsystem2/MATLAB Function ==
  data: u input; y output
function y = fcn(u)

if(u<=0.5)
    y=1;
elseif ((0.5<u)&&(u<3))
    y=(6/5)*(1-u/3);
else
    y=0;
end

== matlab function xobserver/Subsystem2/MATLAB Function1 ==
  data: u input; y output
function y = fcn(u)

if(u<=0.5)
    y=1;
elseif ((0.5<u)&&(u<3))
    y=(6/5)*(1-u/3);
else
    y=0;
end

== matlab function xobserver/Subsystem2/MATLAB Function2 ==
  data: u input; y output
function y = fcn(u)

if(u<=0.5)
    y=1;
elseif ((0.5<u)&&(u<3))
    y=(6/5)*(1-u/3);
else
    y=0;
end

== matlab function xobserver/Subsystem2/MATLAB Function3 ==
  data: u input; y output
function y = fcn(u)

if(u<=0.5)
    y=1;
elseif ((0.5<u)&&(u<3))
    y=(6/5)*(1-u/3);
else
    y=0;
end

== matlab function xobserver/Subsystem2/MATLAB Function4 ==
  data: u input; y output
function y = fcn(u)

if(u<=0.5)
    y=1;
elseif ((0.5<u)&&(u<3))
    y=(6/5)*(1-u/3);
else
    y=0;
end

== matlab function xobserver/Subsystem2/MATLAB Function5 ==
  data: u input; y output
function y = fcn(u)

if(u<=0.5)
    y=1;
elseif ((0.5<u)&&(u<3))
    y=(6/5)*(1-u/3);
else
    y=0;
end

== matlab function xobserver/Subsystem2/MATLAB Function6 ==
  data: u1 input; y output; u2 input
function y = fcn(u1, u2)

y=(u1+u2)/2;

== matlab function xobserver/Subsystem2/MATLAB Function7 ==
  data: u1 input; y output; u2 input
function y = fcn(u1, u2)

y=(u1+u2)/2;

== matlab function xobserver/Subsystem2/MATLAB Function8 ==
  data: u1 input; y output; u2 input
function y = fcn(u1, u2)

y=(u1+u2)/2;

== matlab function xobserver/Subsystem2/MATLAB Function9 ==
  data: u1 input; y output; u2 input
function y = fcn(u1, u2)

y=(u1+u2)/2;

== matlab function xobserver/Subsystem2/MATLAB Function10 ==
  data: u1 input; y output; u2 input
function y = fcn(u1, u2)

y=(u1+u2)/2;

== matlab function xobserver/Subsystem2/MATLAB Function11 ==
  data: u1 input; y output; u2 input
function y = fcn(u1, u2)

y=(u1+u2)/2;

== matlab function xobserver/Subsystem2/MATLAB Function12 ==
  data: u1 input; y output; u2 input; u3 input; x1 input; x2 input; x3 input
function y = fcn(u1, u2, u3, x1, x2, x3)

y = (u1*x1 + u2*x2 + u3*x3)/(u1+u2+u3);

== matlab function xobserver/Subsystem2/MATLAB Function13 ==
  data: u1 input; y output; u2 input; u3 input; x1 input; x2 input; x3 input
function y = fcn(u1, u2, u3, x1, x2, x3)

y = (u1*x1 + u2*x2 + u3*x3)/(u1+u2+u3);

== matlab function xobserver/Subsystem2/MATLAB Function14 ==
  data: u input; y output
function y = fcn(u)

if(u<=0.5)
    y=1;
elseif ((0.5<u)&&(u<3))
    y=(6/5)*(1-u/3);
else
    y=0;
end

== matlab function xobserver/Subsystem2/MATLAB Function15 ==
  data: u input; y output
function y = fcn(u)

if(u<=0.5)
    y=1;
elseif ((0.5<u)&&(u<3))
    y=(6/5)*(1-u/3);
else
    y=0;
end

== matlab function xobserver/Subsystem2/MATLAB Function16 ==
  data: u1 input; y output; u2 input; u3 input; x1 input; x2 input; x3 input
function y = fcn(u1, u2, u3, x1, x2, x3)

y = (u1*x1 + u2*x2 + u3*x3)/(u1+u2+u3);

== matlab function xobserver/Subsystem2/MATLAB Function17 ==
  data: u input; y output
function y = fcn(u)

if(u<=0.5)
    y=1;
elseif ((0.5<u)&&(u<3))
    y=(6/5)*(1-u/3);
else
    y=0;
end

== matlab function xobserver/Subsystem2/MATLAB Function18 ==
  data: u1 input; y output; u2 input
function y = fcn(u1, u2)

y=(u1+u2)/2;

== matlab function xobserver/Subsystem2/MATLAB Function19 ==
  data: u1 input; y output; u2 input
function y = fcn(u1, u2)

y=(u1+u2)/2;

== matlab function xobserver/Subsystem2/MATLAB Function20 ==
  data: u1 input; y output; u2 input
function y = fcn(u1, u2)

y=(u1+u2)/2;

== matlab function xobserver/Observer /Subsystem/MATLAB Function ==
  data: zdhat input; dzhat output; lambda1z input; errorz input
function dzhat = fcn(zdhat, lambda1z, errorz)

dzhat = zdhat + lambda1z*power(abs(errorz),1/2)*sign(errorz);
%%dxhat = xdhat;

== matlab function xobserver/Observer /Subsystem/MATLAB Function1 ==
  data: lambda2z input; dzdhat output; errorz input; roll input; pitch input; ut input
function dzdhat = fcn(lambda2z, errorz, roll, pitch, ut)

dzdhat = lambda2z*sign(errorz) + (cos(roll)*cos(pitch))*ut/1.653 - 9.81;
%%dzdhat = (cos(roll)*cos(pitch))*ut/1.653 - 9.81;

== matlab function xobserver/Subsystem2/MATLAB Function21 ==
  data: u input; y output
function y = fcn(u)

if(u<=0.2)
    y=1;
elseif ((0.2<u)&&(u<1.2))
    y=(6/5)*(1-u/1.2);
else
    y=0;
end

== matlab function xobserver/Subsystem2/MATLAB Function22 ==
  data: u input; y output
function y = fcn(u)

if(u<=0.2)
    y=1;
elseif ((0.2<u)&&(u<1.2))
    y=(6/5)*(1-u/1.2);
else
    y=0;
end

== matlab function xobserver/Subsystem2/MATLAB Function23 ==
  data: u1 input; y output; u2 input; u3 input; x1 input; x2 input; x3 input
function y = fcn(u1, u2, u3, x1, x2, x3)

y = (u1*x1 + u2*x2 + u3*x3)/(u1+u2+u3);

== matlab function xobserver/Subsystem2/MATLAB Function24 ==
  data: u input; y output
function y = fcn(u)

if(u<=0.2)
    y=1;
elseif ((0.2<u)&&(u<1.2))
    y=(6/5)*(1-u/1.2);
else
    y=0;
end

== matlab function xobserver/Subsystem2/MATLAB Function25 ==
  data: u1 input; y output; u2 input
function y = fcn(u1, u2)

y=(u1+u2)/2;

== matlab function xobserver/Subsystem2/MATLAB Function26 ==
  data: u1 input; y output; u2 input
function y = fcn(u1, u2)

y=(u1+u2)/2;

== matlab function xobserver/Subsystem2/MATLAB Function27 ==
  data: u1 input; y output; u2 input
function y = fcn(u1, u2)

y=(u1+u2)/2;

== matlab function xobserver/Subsystem2/Add for recovery ==
  data: u1 input; y output; u2 input; u3 input; u4 input
function y = fcn(u1,u2,u3,u4)

if(u4 == 0)
    y=u1;
else
    y=(u2+u3)/2;
end

== matlab function xobserver/Subsystem2/Add for recovery1 ==
  data: u1 input; y output; u2 input; u3 input
function y = time_of_fault(u1,u2,u3)

if(u1==0 && u2==0)
    y=u3;
else
    y=0;
end

== matlab function xobserver/Subsystem2/Add for recovery2 ==
  data: u1 input; y output; u2 input; u3 input
function y = time_of_fault(u1,u2,u3)

if(u1==0 && u2==0)
    y=u3;
else
    y=0;
end

== matlab function xobserver/Subsystem2/Add for recovery3 ==
  data: u1 input; y output; u2 input; u3 input; u4 input
function y = fcn(u1,u2,u3,u4)

if(u4 == 0)
    y=u1;
else
    y=(u2+u3)/2;
end

== matlab function xobserver/Subsystem2/Add for recovery4 ==
  data: u1 input; y output; u2 input; u3 input; u4 input
function y = fcn(u1,u2,u3,u4)

if(u4 == 0)
    y=u1;
else
    y=(u2+u3)/2;
end

== matlab function xobserver/Subsystem2/Add for recovery5 ==
  data: u1 input; y output; u2 input; u3 input
function y = time_of_fault(u1,u2,u3)

if(u1==0 && u2==0)
    y=u3;
else
    y=0;
end
